simulink model "case9"  (R2024b)
settings: Solver=FixedStepAuto  StartTime=0  StopTime=1  FixedStep=1e-7  RelTol=1e-3
values from neighbouring files (symbols this model uses):
  SG_D_1_D = 0.01056    [IEEE9_case_parameters.m]    (also in case1_parameters.m; case2_parameters.m; case3_parameters.m; case4_parameters.m)
  SG_D_1_EnableSaturation = 0    [IEEE9_case_parameters.m]    (also in case1_parameters.m; case2_parameters.m; case3_parameters.m; case4_parameters.m)
  SG_D_1_f0 = 60    [IEEE9_case_parameters.m]    (also in case1_parameters.m; case2_parameters.m; case3_parameters.m; case4_parameters.m)
  SG_D_1_H = 7.5    [IEEE9_case_parameters.m]    (also in case1_parameters.m; case2_parameters.m; case3_parameters.m; case4_parameters.m)
  SG_D_1_K_A = 20    [IEEE9_case_parameters.m]    (also in case1_parameters.m; case2_parameters.m; case3_parameters.m; case4_parameters.m)
  SG_D_1_K_E = 1.000000e+1    (= 10)    [IEEE9_case_parameters.m]    (also in case1_parameters.m; case2_parameters.m; case3_parameters.m; case4_parameters.m)
  SG_D_1_K_F = 2.363    [IEEE9_case_parameters.m]    (also in case1_parameters.m; case2_parameters.m; case3_parameters.m; case4_parameters.m)
  SG_D_1_K_s = 0.5    [IEEE9_case_parameters.m]    (also in case1_parameters.m = 5; case2_parameters.m = 5; case3_parameters.m = 5; case4_parameters.m = 5)
  SG_D_1_R_a = 0.001088    [IEEE9_case_parameters.m]    (also in case1_parameters.m; case2_parameters.m; case3_parameters.m; case4_parameters.m)
  SG_D_1_S_A = 1    [IEEE9_case_parameters.m]    (also in case1_parameters.m; case2_parameters.m; case3_parameters.m; case4_parameters.m)
  SG_D_1_S_B = 0.103    [IEEE9_case_parameters.m]    (also in case1_parameters.m; case2_parameters.m; case3_parameters.m; case4_parameters.m)
  SG_D_1_S_N = 10.659857    [IEEE9_case_parameters.m]    (also in case1_parameters.m; case2_parameters.m; case3_parameters.m; case4_parameters.m)
  SG_D_1_SpeedPara = 200    [IEEE9_case_parameters.m]    (also in case1_parameters.m; case2_parameters.m; case3_parameters.m; case4_parameters.m)
  SG_D_1_T_0 = 0.720173    [IEEE9_case_parameters.m]    (also in case1_parameters.m = 0.755522; case2_parameters.m = 0.808931; case3_parameters.m = 0.869402; case4_parameters.m = 0.729316)
  SG_D_1_T_1 = 0.3    [IEEE9_case_parameters.m]    (also in case1_parameters.m; case2_parameters.m; case3_parameters.m; case4_parameters.m)
  SG_D_1_T_2 = 0.05    [IEEE9_case_parameters.m]    (also in case1_parameters.m; case2_parameters.m; case3_parameters.m; case4_parameters.m)
  SG_D_1_T_3 = 0.02    [IEEE9_case_parameters.m]    (also in case1_parameters.m; case2_parameters.m; case3_parameters.m; case4_parameters.m)
  SG_D_1_T_4 = 0.005    [IEEE9_case_parameters.m]    (also in case1_parameters.m; case2_parameters.m; case3_parameters.m; case4_parameters.m)
  SG_D_1_T_A = 0.02    [IEEE9_case_parameters.m]    (also in case1_parameters.m; case2_parameters.m; case3_parameters.m; case4_parameters.m)
  SG_D_1_T_dd = 8.000000e+0    (= 8)    [IEEE9_case_parameters.m]    (also in case1_parameters.m; case2_parameters.m; case3_parameters.m; case4_parameters.m)
  SG_D_1_T_ddd = 0.04    [IEEE9_case_parameters.m]    (also in case1_parameters.m; case2_parameters.m; case3_parameters.m; case4_parameters.m)
  SG_D_1_T_E = 0.314    [IEEE9_case_parameters.m]    (also in case1_parameters.m; case2_parameters.m; case3_parameters.m; case4_parameters.m)
  SG_D_1_T_F = 0.35    [IEEE9_case_parameters.m]    (also in case1_parameters.m; case2_parameters.m; case3_parameters.m; case4_parameters.m)
  SG_D_1_T_qd = 0.8    [IEEE9_case_parameters.m]    (also in case1_parameters.m; case2_parameters.m; case3_parameters.m; case4_parameters.m)
  SG_D_1_T_qdd = 0.02    [IEEE9_case_parameters.m]    (also in case1_parameters.m; case2_parameters.m; case3_parameters.m; case4_parameters.m)
  SG_D_1_T_speed = 0.1    [IEEE9_case_parameters.m]    (also in case1_parameters.m = 200; case2_parameters.m = 200; case3_parameters.m = 200; case4_parameters.m = 200)
  SG_D_1_T_w = 0.5    [IEEE9_case_parameters.m]    (also in case1_parameters.m; case2_parameters.m; case3_parameters.m; case4_parameters.m)
  SG_D_1_V_ref = 1.990276    [IEEE9_case_parameters.m]    (also in case1_parameters.m = 2.042296; case2_parameters.m = 2.051388; case3_parameters.m = 2.089584; case4_parameters.m = 2.01845)
  SG_D_1_w_ref = 376.991118    [IEEE9_case_parameters.m]    (also in case1_parameters.m; case2_parameters.m; case3_parameters.m; case4_parameters.m)
  SG_D_1_wb = 6.000000e+1    (= 60)    [IEEE9_case_parameters.m]    (also in case1_parameters.m; case2_parameters.m; case3_parameters.m; case4_parameters.m)
  SG_D_1_x_d = 1.9    [IEEE9_case_parameters.m]    (also in case1_parameters.m; case2_parameters.m; case3_parameters.m; case4_parameters.m)
  SG_D_1_x_dd = 0.302    [IEEE9_case_parameters.m]    (also in case1_parameters.m; case2_parameters.m; case3_parameters.m; case4_parameters.m)
  SG_D_1_x_ddd = 0.204    [IEEE9_case_parameters.m]    (also in case1_parameters.m; case2_parameters.m; case3_parameters.m; case4_parameters.m)
  SG_D_1_x_l = 0.05    [IEEE9_case_parameters.m]    (also in case1_parameters.m; case2_parameters.m; case3_parameters.m; case4_parameters.m)
  SG_D_1_x_q = 1.3    [IEEE9_case_parameters.m]    (also in case1_parameters.m; case2_parameters.m; case3_parameters.m; case4_parameters.m)
  SG_D_1_x_qd = 0.5    [IEEE9_case_parameters.m]    (also in case1_parameters.m; case2_parameters.m; case3_parameters.m; case4_parameters.m)
  SG_D_1_x_qdd = 0.3    [IEEE9_case_parameters.m]    (also in case1_parameters.m; case2_parameters.m; case3_parameters.m; case4_parameters.m)
  SG_D_2_D = 0.02    [IEEE9_case_parameters.m]    (also in case1_parameters.m; case2_parameters.m; case3_parameters.m; case4_parameters.m)
  SG_D_2_EnableSaturation = 0    [IEEE9_case_parameters.m]    (also in case1_parameters.m; case2_parameters.m; case3_parameters.m; case4_parameters.m)
  SG_D_2_f0 = 60    [IEEE9_case_parameters.m]    (also in case1_parameters.m; case2_parameters.m; case3_parameters.m; case4_parameters.m)
  SG_D_2_H = 8.000000e+0    (= 8)    [IEEE9_case_parameters.m]    (also in case1_parameters.m; case2_parameters.m; case3_parameters.m; case4_parameters.m)
  SG_D_2_K_A = 20    [IEEE9_case_parameters.m]    (also in case1_parameters.m; case2_parameters.m; case3_parameters.m; case4_parameters.m)
  SG_D_2_K_E = 1.000000e+1    (= 10)    [IEEE9_case_parameters.m]    (also in case1_parameters.m; case2_parameters.m; case3_parameters.m; case4_parameters.m)
  SG_D_2_K_F = 2.363    [IEEE9_case_parameters.m]    (also in case1_parameters.m; case2_parameters.m; case3_parameters.m; case4_parameters.m)
  SG_D_2_K_s = 0.5    [IEEE9_case_parameters.m]    (also in case1_parameters.m = 4; case2_parameters.m = 4; case3_parameters.m = 4; case4_parameters.m = 4)
  SG_D_2_R_a = 0.001088    [IEEE9_case_parameters.m]    (also in case1_parameters.m; case2_parameters.m; case3_parameters.m; case4_parameters.m)
  SG_D_2_S_A = 1    [IEEE9_case_parameters.m]    (also in case1_parameters.m; case2_parameters.m; case3_parameters.m; case4_parameters.m)
  SG_D_2_S_B = 0.103    [IEEE9_case_parameters.m]    (also in case1_parameters.m; case2_parameters.m; case3_parameters.m; case4_parameters.m)
  SG_D_2_S_N = 10.659857    [IEEE9_case_parameters.m]    (also in case1_parameters.m; case2_parameters.m; case3_parameters.m; case4_parameters.m)
  SG_D_2_SpeedPara = 200    [IEEE9_case_parameters.m]    (also in case1_parameters.m; case2_parameters.m; case3_parameters.m; case4_parameters.m)
  SG_D_2_T_0 = 1.632913    [IEEE9_case_parameters.m]    (also in case1_parameters.m = 1.632925; case2_parameters.m = 1.632915; case3_parameters.m = 1.632914; case4_parameters.m = 1.632927)
  SG_D_2_T_1 = 0.2    [IEEE9_case_parameters.m]    (also in case1_parameters.m; case2_parameters.m; case3_parameters.m; case4_parameters.m)
  SG_D_2_T_2 = 0.05    [IEEE9_case_parameters.m]    (also in case1_parameters.m; case2_parameters.m; case3_parameters.m; case4_parameters.m)
  SG_D_2_T_3 = 0.02    [IEEE9_case_parameters.m]    (also in case1_parameters.m; case2_parameters.m; case3_parameters.m; case4_parameters.m)
  SG_D_2_T_4 = 0.005    [IEEE9_case_parameters.m]    (also in case1_parameters.m; case2_parameters.m; case3_parameters.m; case4_parameters.m)
  SG_D_2_T_A = 0.02    [IEEE9_case_parameters.m]    (also in case1_parameters.m; case2_parameters.m; case3_parameters.m; case4_parameters.m)
  SG_D_2_T_dd = 7.9    [IEEE9_case_parameters.m]    (also in case1_parameters.m; case2_parameters.m; case3_parameters.m; case4_parameters.m)
  SG_D_2_T_ddd = 0.04    [IEEE9_case_parameters.m]    (also in case1_parameters.m; case2_parameters.m; case3_parameters.m; case4_parameters.m)
  SG_D_2_T_E = 0.314    [IEEE9_case_parameters.m]    (also in case1_parameters.m; case2_parameters.m; case3_parameters.m; case4_parameters.m)
  SG_D_2_T_F = 0.35    [IEEE9_case_parameters.m]    (also in case1_parameters.m; case2_parameters.m; case3_parameters.m; case4_parameters.m)
  SG_D_2_T_qd = 0.8    [IEEE9_case_parameters.m]    (also in case1_parameters.m; case2_parameters.m; case3_parameters.m; case4_parameters.m)
  SG_D_2_T_qdd = 0.015    [IEEE9_case_parameters.m]    (also in case1_parameters.m; case2_parameters.m; case3_parameters.m; case4_parameters.m)
  SG_D_2_T_speed = 0.1    [IEEE9_case_parameters.m]    (also in case1_parameters.m = 150; case2_parameters.m = 150; case3_parameters.m = 150; case4_parameters.m = 150)
  SG_D_2_T_w = 0.35    [IEEE9_case_parameters.m]    (also in case1_parameters.m; case2_parameters.m; case3_parameters.m; case4_parameters.m)
  SG_D_2_V_ref = 2.58547    [IEEE9_case_parameters.m]    (also in case1_parameters.m = 2.597896; case2_parameters.m = 2.587136; case3_parameters.m = 2.586042; case4_parameters.m = 2.599679)
  SG_D_2_w_ref = 376.991118    [IEEE9_case_parameters.m]    (also in case1_parameters.m; case2_parameters.m; case3_parameters.m; case4_parameters.m)
  SG_D_2_wb = 6.000000e+1    (= 60)    [IEEE9_case_parameters.m]    (also in case1_parameters.m; case2_parameters.m; case3_parameters.m; case4_parameters.m)
  SG_D_2_x_d = 1.8    [IEEE9_case_parameters.m]    (also in case1_parameters.m; case2_parameters.m; case3_parameters.m; case4_parameters.m)
  SG_D_2_x_dd = 0.302    [IEEE9_case_parameters.m]    (also in case1_parameters.m; case2_parameters.m; case3_parameters.m; case4_parameters.m)
  SG_D_2_x_ddd = 0.204    [IEEE9_case_parameters.m]    (also in case1_parameters.m; case2_parameters.m; case3_parameters.m; case4_parameters.m)
  SG_D_2_x_l = 0.05    [IEEE9_case_parameters.m]    (also in case1_parameters.m; case2_parameters.m; case3_parameters.m; case4_parameters.m)
  SG_D_2_x_q = 1.25    [IEEE9_case_parameters.m]    (also in case1_parameters.m; case2_parameters.m; case3_parameters.m; case4_parameters.m)
  SG_D_2_x_qd = 0.5    [IEEE9_case_parameters.m]    (also in case1_parameters.m; case2_parameters.m; case3_parameters.m; case4_parameters.m)
  SG_D_2_x_qdd = 0.3    [IEEE9_case_parameters.m]    (also in case1_parameters.m; case2_parameters.m; case3_parameters.m; case4_parameters.m)
  SG_D_3_D = 0.02    [IEEE9_case_parameters.m]    (also in case1_parameters.m; case2_parameters.m; case3_parameters.m; case4_parameters.m)
  SG_D_3_EnableSaturation = 0    [IEEE9_case_parameters.m]    (also in case1_parameters.m; case2_parameters.m; case3_parameters.m; case4_parameters.m)
  SG_D_3_f0 = 60    [IEEE9_case_parameters.m]    (also in case1_parameters.m; case2_parameters.m; case3_parameters.m; case4_parameters.m)
  SG_D_3_H = 7.7    [IEEE9_case_parameters.m]    (also in case1_parameters.m; case2_parameters.m; case3_parameters.m; case4_parameters.m)
  SG_D_3_K_A = 20    [IEEE9_case_parameters.m]    (also in case1_parameters.m; case2_parameters.m; case3_parameters.m; case4_parameters.m)
  SG_D_3_K_E = 1.000000e+1    (= 10)    [IEEE9_case_parameters.m]    (also in case1_parameters.m; case2_parameters.m; case3_parameters.m; case4_parameters.m)
  SG_D_3_K_F = 2.363    [IEEE9_case_parameters.m]    (also in case1_parameters.m; case2_parameters.m; case3_parameters.m; case4_parameters.m)
  SG_D_3_K_s = 0.2    [IEEE9_case_parameters.m]    (also in case1_parameters.m = 2; case2_parameters.m = 2; case3_parameters.m = 2; case4_parameters.m = 2)
  SG_D_3_R_a = 0.001088    [IEEE9_case_parameters.m]    (also in case1_parameters.m; case2_parameters.m; case3_parameters.m; case4_parameters.m)
  SG_D_3_S_A = 1    [IEEE9_case_parameters.m]    (also in case1_parameters.m; case2_parameters.m; case3_parameters.m; case4_parameters.m)
  SG_D_3_S_B = 0.103    [IEEE9_case_parameters.m]    (also in case1_parameters.m; case2_parameters.m; case3_parameters.m; case4_parameters.m)
  SG_D_3_S_N = 10.659857    [IEEE9_case_parameters.m]    (also in case1_parameters.m; case2_parameters.m; case3_parameters.m; case4_parameters.m)
  SG_D_3_SpeedPara = 200    [IEEE9_case_parameters.m]    (also in case1_parameters.m; case2_parameters.m; case3_parameters.m; case4_parameters.m)
  SG_D_3_T_0 = 0.850788    [IEEE9_case_parameters.m]    (also in case1_parameters.m = 0.850786; case2_parameters.m = 0.850787; case3_parameters.m; case4_parameters.m = 0.850786)
  SG_D_3_T_1 = 0.2    [IEEE9_case_parameters.m]    (also in case1_parameters.m; case2_parameters.m; case3_parameters.m; case4_parameters.m)
  SG_D_3_T_2 = 0.05    [IEEE9_case_parameters.m]    (also in case1_parameters.m; case2_parameters.m; case3_parameters.m; case4_parameters.m)
  SG_D_3_T_3 = 0.02    [IEEE9_case_parameters.m]    (also in case1_parameters.m; case2_parameters.m; case3_parameters.m; case4_parameters.m)
  SG_D_3_T_4 = 0.005    [IEEE9_case_parameters.m]    (also in case1_parameters.m; case2_parameters.m; case3_parameters.m; case4_parameters.m)
  SG_D_3_T_A = 0.02    [IEEE9_case_parameters.m]    (also in case1_parameters.m; case2_parameters.m; case3_parameters.m; case4_parameters.m)
  SG_D_3_T_dd = 8.1    [IEEE9_case_parameters.m]    (also in case1_parameters.m; case2_parameters.m; case3_parameters.m; case4_parameters.m)
  SG_D_3_T_ddd = 0.04    [IEEE9_case_parameters.m]    (also in case1_parameters.m; case2_parameters.m; case3_parameters.m; case4_parameters.m)
  SG_D_3_T_E = 0.314    [IEEE9_case_parameters.m]    (also in case1_parameters.m; case2_parameters.m; case3_parameters.m; case4_parameters.m)
  SG_D_3_T_F = 0.35    [IEEE9_case_parameters.m]    (also in case1_parameters.m; case2_parameters.m; case3_parameters.m; case4_parameters.m)
  SG_D_3_T_qd = 0.8    [IEEE9_case_parameters.m]    (also in case1_parameters.m; case2_parameters.m; case3_parameters.m; case4_parameters.m)
  SG_D_3_T_qdd = 0.015    [IEEE9_case_parameters.m]    (also in case1_parameters.m; case2_parameters.m; case3_parameters.m; case4_parameters.m)
  SG_D_3_T_speed = 0.1    [IEEE9_case_parameters.m]    (also in case1_parameters.m = 180; case2_parameters.m = 180; case3_parameters.m = 180; case4_parameters.m = 180)
  SG_D_3_T_w = 0.4    [IEEE9_case_parameters.m]    (also in case1_parameters.m; case2_parameters.m; case3_parameters.m; case4_parameters.m)
  SG_D_3_V_ref = 1.892727    [IEEE9_case_parameters.m]    (also in case1_parameters.m = 1.906439; case2_parameters.m = 1.895535; case3_parameters.m = 1.892105; case4_parameters.m = 1.906598)
  SG_D_3_w_ref = 376.991118    [IEEE9_case_parameters.m]    (also in case1_parameters.m; case2_parameters.m; case3_parameters.m; case4_parameters.m)
  SG_D_3_wb = 6.000000e+1    (= 60)    [IEEE9_case_parameters.m]    (also in case1_parameters.m; case2_parameters.m; case3_parameters.m; case4_parameters.m)
  SG_D_3_x_d = 1.85    [IEEE9_case_parameters.m]    (also in case1_parameters.m; case2_parameters.m; case3_parameters.m; case4_parameters.m)
  SG_D_3_x_dd = 0.302    [IEEE9_case_parameters.m]    (also in case1_parameters.m; case2_parameters.m; case3_parameters.m; case4_parameters.m)
  SG_D_3_x_ddd = 0.204    [IEEE9_case_parameters.m]    (also in case1_parameters.m; case2_parameters.m; case3_parameters.m; case4_parameters.m)
  SG_D_3_x_l = 0.05    [IEEE9_case_parameters.m]    (also in case1_parameters.m; case2_parameters.m; case3_parameters.m; case4_parameters.m)
  SG_D_3_x_q = 1.2    [IEEE9_case_parameters.m]    (also in case1_parameters.m; case2_parameters.m; case3_parameters.m; case4_parameters.m)
  SG_D_3_x_qd = 0.5    [IEEE9_case_parameters.m]    (also in case1_parameters.m; case2_parameters.m; case3_parameters.m; case4_parameters.m)
  SG_D_3_x_qdd = 0.3    [IEEE9_case_parameters.m]    (also in case1_parameters.m; case2_parameters.m; case3_parameters.m; case4_parameters.m)
(part 7 of 12)

== system case9/Apparatus/SG_D_1/i_q_SG_D_1_block ==
  note: i_q_SG_D_1 in case9
      | $-\frac{\sin\left(\theta _{\mathrm{SG},D,1}\right)\,\left(\psi _{q,\mathrm{SG},D,1}+\frac{\psi _{\mathrm{gq},\mathrm{SG},D,1}\,\left(x_{l}-x_{\mathrm{qdd}}\right)}{x_{l}-x_{\mathrm{qd}}}+\frac{\psi _{\mathrm{kq},\mathrm{SG},D,1}\,\left(x_{\mathrm{qd}}-x_{\mathrm{qdd}}\right)}{x_{l}-x_{\mathrm{qd}}}\right)}{x_{\mathrm{qdd}}}-\frac{\cos\left(\theta _{\mathrm{SG},D,1}\right)\,\left(\frac{\psi _{\mathrm{1d},\mathrm{SG},D,1}\,\left(x_{\mathrm{dd}}-x_{\mathrm{ddd}}\right)}{x_{\mathrm{dd}}-x_{l}}-\psi _{d,\mathrm{SG},D,1}+\frac{\psi _{\mathrm{fd},\mathrm{SG},D,1}\,\left(x_{\mathrm{ddd}}-x_{l}\right)}{x_{\mathrm{dd}}-x_{l}}\right)}{x_{\mathrm{ddd}}}$
      | Automatically generated on 2025-10-31 19:34:49 .
  State_psi_gq_SG_D_1_092c5 : Inport
  State_psi_kq_SG_D_1_97f5f : Inport  Port=2
  State_psi_q_SG_D_1_fdadd : Inport  Port=3
  State_theta_SG_D_1_3c1fa : Inport  Port=4
  State_psi_1d_SG_D_1_7b40d : Inport  Port=5
  State_psi_d_SG_D_1_0e386 : Inport  Port=6
  State_psi_fd_SG_D_1_9fe64 : Inport  Port=7
  State_theta_SG_D_1_71fb6 : Inport  Port=8
  Add_0017d : Sum
  Add_35a64 : Sum
  Add_56630 : Sum
  Add_62db7 : Sum
  Add_95d78 : Sum
  Add_e1f2e : Sum
  Constant_-1_14a26 : Constant  Value=-1
  Constant_-1_1cd36 : Constant  Value=-1
  Constant_-1_24052 : Constant  Value=-1
  Constant_-1_72e90 : Constant  Value=-1
  Constant_-1_8fd2e : Constant  Value=-1
  Constant_x_dd_843a6 : Constant  Value=x_dd
  Constant_x_dd_8e74f : Constant  Value=x_dd
  Constant_x_dd_e3151 : Constant  Value=x_dd
  Constant_x_ddd_51e8b : Constant  Value=x_ddd
  Constant_x_ddd_cca8e : Constant  Value=x_ddd
  Constant_x_ddd_d6eda : Constant  Value=x_ddd
  Constant_x_l_3e9e8 : Constant  Value=x_l
  Constant_x_l_9dea0 : Constant  Value=x_l
  Constant_x_l_a6233 : Constant  Value=x_l
  Constant_x_l_c84a1 : Constant  Value=x_l
  Constant_x_l_c867c : Constant  Value=x_l
  Constant_x_l_f552f : Constant  Value=x_l
  Constant_x_qd_56b92 : Constant  Value=x_qd
  Constant_x_qd_58631 : Constant  Value=x_qd
  Constant_x_qd_adad9 : Constant  Value=x_qd
  Constant_x_qdd_01789 : Constant  Value=x_qdd
  Constant_x_qdd_72f85 : Constant  Value=x_qdd
  Constant_x_qdd_ff6ca : Constant  Value=x_qdd
  Divide_65d14 : Product  Inputs=*/
  Divide_84916 : Product  Inputs=*/
  Divide_a2796 : Product  Inputs=*/
  Divide_a496a : Product  Inputs=*/
  Divide_bf3d1 : Product  Inputs=*/
  Divide_d6104 : Product  Inputs=*/
  MathFunc_cos_5e1d4 : Trigonometry  Operator=cos
  MathFunc_sin_468db : Trigonometry
  Product_13cd1 : Product
  Product_232ad : Product
  Product_41f3d : Product
  Product_456f6 : Product
  Product_4694f : Product
  Product_4cb2c : Product
  Product_83cb5 : Product
  Product_a6406 : Product
  Product_a9c33 : Product
  Product_d6079 : Product
  Product_f9405 : Product
  Subtract_3022c : Sum  Inputs=+-
  Subtract_3886e : Sum  Inputs=+-
  Subtract_5dabf : Sum  Inputs=+-
  Subtract_96f7c : Sum  Inputs=+-
  Subtract_9b1aa : Sum  Inputs=+-
  Subtract_e0046 : Sum  Inputs=+-
  Subtract_ea4b7 : Sum  Inputs=+-
  Blockout_i_q_SG_D_1_cd846 : Outport
  wires:
  State_theta_SG_D_1_71fb6/1 -> MathFunc_cos_5e1d4/1
  State_psi_fd_SG_D_1_9fe64/1 -> Product_f9405/1
  Constant_-1_72e90/1 -> Product_a6406/1
  Constant_x_l_c867c/1 -> Product_a6406/2
  Subtract_5dabf/1 -> Product_f9405/2
  Constant_x_l_9dea0/1 -> Subtract_9b1aa/2
  Product_a6406/1 -> Add_0017d/1
  Constant_x_qdd_ff6ca/1 -> Add_0017d/2
  Constant_x_qd_adad9/1 -> Subtract_e0046/1
  Constant_x_qdd_72f85/1 -> Divide_65d14/2
  MathFunc_sin_468db/1 -> Product_13cd1/2
  Constant_-1_8fd2e/1 -> Product_83cb5/1
  Constant_x_qdd_01789/1 -> Subtract_e0046/2
  Add_56630/1 -> Product_4694f/2
  Product_456f6/1 -> Divide_84916/1
  Constant_x_l_f552f/1 -> Product_83cb5/2
  Constant_-1_14a26/1 -> Product_232ad/1
  Constant_x_l_3e9e8/1 -> Product_232ad/2
  State_psi_gq_SG_D_1_092c5/1 -> Product_456f6/1
  Add_0017d/1 -> Product_456f6/2
  Divide_a496a/1 -> Add_e1f2e/1
  Product_83cb5/1 -> Add_35a64/1
  Divide_65d14/1 -> Add_95d78/1
  Constant_x_qd_56b92/1 -> Add_35a64/2
  State_psi_kq_SG_D_1_97f5f/1 -> Product_4cb2c/1
  Add_e1f2e/1 -> Subtract_96f7c/1
  Subtract_e0046/1 -> Product_4cb2c/2
  Divide_84916/1 -> Subtract_3022c/1
  Add_35a64/1 -> Divide_84916/2
  Product_232ad/1 -> Add_62db7/1
  Constant_x_qd_58631/1 -> Add_62db7/2
  Constant_-1_1cd36/1 -> Product_a9c33/1
  MathFunc_cos_5e1d4/1 -> Product_d6079/2
  Product_f9405/1 -> Divide_d6104/1
  State_psi_1d_SG_D_1_7b40d/1 -> Product_a9c33/2
  Constant_x_l_c84a1/1 -> Subtract_3886e/2
  Constant_x_dd_e3151/1 -> Subtract_ea4b7/1
  Divide_d6104/1 -> Subtract_96f7c/2
  Constant_x_ddd_d6eda/1 -> Subtract_ea4b7/2
  Product_d6079/1 -> Divide_bf3d1/1
  Product_4cb2c/1 -> Divide_a2796/1
  Product_a9c33/1 -> Product_41f3d/1
  Add_62db7/1 -> Divide_a2796/2
  Subtract_ea4b7/1 -> Product_41f3d/2
  State_psi_d_SG_D_1_0e386/1 -> Add_e1f2e/2
  Constant_x_dd_8e74f/1 -> Subtract_9b1aa/1
  Constant_x_ddd_cca8e/1 -> Subtract_5dabf/1
  Constant_x_l_a6233/1 -> Subtract_5dabf/2
  Divide_bf3d1/1 -> Add_95d78/2
  Divide_a2796/1 -> Subtract_3022c/2
  State_theta_SG_D_1_3c1fa/1 -> MathFunc_sin_468db/1
  Product_41f3d/1 -> Divide_a496a/1
  Subtract_9b1aa/1 -> Divide_a496a/2
  Constant_x_dd_843a6/1 -> Subtract_3886e/1
  Subtract_3022c/1 -> Add_56630/1
  State_psi_q_SG_D_1_fdadd/1 -> Add_56630/2
  Subtract_3886e/1 -> Divide_d6104/2
  Subtract_96f7c/1 -> Product_d6079/1
  Constant_-1_24052/1 -> Product_4694f/1
  Product_4694f/1 -> Product_13cd1/1
  Product_13cd1/1 -> Divide_65d14/1
  Constant_x_ddd_51e8b/1 -> Divide_bf3d1/2
  Add_95d78/1 -> Blockout_i_q_SG_D_1_cd846/1

== system case9/Apparatus/SG_D_1/theta_SG_D_1_out_block ==
  note: theta_SG_D_1_out in case9
      | $\theta _{\mathrm{SG},D,1}$
      | Automatically generated on 2025-10-31 19:34:50 .
  State_theta_SG_D_1_b223f : Inport
  Blockout_theta_SG_D_1_out_ac5bf : Outport
  wires:
  State_theta_SG_D_1_b223f/1 -> Blockout_theta_SG_D_1_out_ac5bf/1

== system case9/Apparatus/SG_D_1/w_SG_D_1_out_block ==
  note: w_SG_D_1_out in case9
      | $w_{\mathrm{SG},D,1}$
      | Automatically generated on 2025-10-31 19:34:50 .
  State_w_SG_D_1_3e49a : Inport
  Blockout_w_SG_D_1_out_45494 : Outport
  wires:
  State_w_SG_D_1_3e49a/1 -> Blockout_w_SG_D_1_out_45494/1

== system case9/Apparatus/SG_D_2/T_e_SG_D_2_block ==
  note: T_e_SG_D_2 in case9
      | $-\frac{\psi _{d,\mathrm{SG},D,2}\,\left(\psi _{q,\mathrm{SG},D,2}+\frac{\psi _{\mathrm{gq},\mathrm{SG},D,2}\,\left(x_{l}-x_{\mathrm{qdd}}\right)}{x_{l}-x_{\mathrm{qd}}}+\frac{\psi _{\mathrm{kq},\mathrm{SG},D,2}\,\left(x_{\mathrm{qd}}-x_{\mathrm{qdd}}\right)}{x_{l}-x_{\mathrm{qd}}}\right)}{x_{\mathrm{qdd}}}-\frac{\psi _{q,\mathrm{SG},D,2}\,\left(\frac{\psi _{\mathrm{1d},\mathrm{SG},D,2}\,\left(x_{\mathrm{dd}}-x_{\mathrm{ddd}}\right)}{x_{\mathrm{dd}}-x_{l}}-\psi _{d,\mathrm{SG},D,2}+\frac{\psi _{\mathrm{fd},\mathrm{SG},D,2}\,\left(x_{\mathrm{ddd}}-x_{l}\right)}{x_{\mathrm{dd}}-x_{l}}\right)}{x_{\mathrm{ddd}}}$
      | Automatically generated on 2025-10-31 19:35:08 .
  State_psi_d_SG_D_2_9606a : Inport
  State_psi_gq_SG_D_2_f0a68 : Inport  Port=2
  State_psi_kq_SG_D_2_17e3d : Inport  Port=3
  State_psi_q_SG_D_2_a73d1 : Inport  Port=4
  State_psi_q_SG_D_2_2dc20 : Inport  Port=5
  State_psi_1d_SG_D_2_dfc50 : Inport  Port=6
  State_psi_d_SG_D_2_7cb77 : Inport  Port=7
  State_psi_fd_SG_D_2_946fe : Inport  Port=8
  Add_0b222 : Sum
  Add_30e81 : Sum
  Add_8b206 : Sum
  Add_d85b4 : Sum
  Add_e0a82 : Sum
  Add_ed19d : Sum
  Constant_-1_3a2ab : Constant  Value=-1
  Constant_-1_81492 : Constant  Value=-1
  Constant_-1_89beb : Constant  Value=-1
  Constant_-1_b1e92 : Constant  Value=-1
  Constant_-1_c9ed8 : Constant  Value=-1
  Constant_x_dd_50243 : Constant  Value=x_dd
  Constant_x_dd_be71b : Constant  Value=x_dd
  Constant_x_dd_dd49a : Constant  Value=x_dd
  Constant_x_ddd_2d22c : Constant  Value=x_ddd
  Constant_x_ddd_b2247 : Constant  Value=x_ddd
  Constant_x_ddd_d3b5a : Constant  Value=x_ddd
  Constant_x_l_1576d : Constant  Value=x_l
  Constant_x_l_72a63 : Constant  Value=x_l
  Constant_x_l_91dea : Constant  Value=x_l
  Constant_x_l_b4de2 : Constant  Value=x_l
  Constant_x_l_bb09d : Constant  Value=x_l
  Constant_x_l_e80c1 : Constant  Value=x_l
  Constant_x_qd_20bdd : Constant  Value=x_qd
  Constant_x_qd_9a586 : Constant  Value=x_qd
  Constant_x_qd_bcee2 : Constant  Value=x_qd
  Constant_x_qdd_146fc : Constant  Value=x_qdd
  Constant_x_qdd_28a0e : Constant  Value=x_qdd
  Constant_x_qdd_c7836 : Constant  Value=x_qdd
  Divide_1415d : Product  Inputs=*/
  Divide_24622 : Product  Inputs=*/
  Divide_4fb71 : Product  Inputs=*/
  Divide_6dd3b : Product  Inputs=*/
  Divide_801a8 : Product  Inputs=*/
  Divide_a4770 : Product  Inputs=*/
  Product_10174 : Product
  Product_280fc : Product
  Product_3044b : Product
  Product_3eab5 : Product
  Product_600d6 : Product
  Product_6735f : Product
  Product_77108 : Product
  Product_78fb9 : Product
  Product_8289b : Product
  Product_dbfcd : Product
  Product_e661d : Product
  Subtract_1d9de : Sum  Inputs=+-
  Subtract_55562 : Sum  Inputs=+-
  Subtract_635aa : Sum  Inputs=+-
  Subtract_661d1 : Sum  Inputs=+-
  Subtract_7ba2e : Sum  Inputs=+-
  Subtract_cacd5 : Sum  Inputs=+-
  Subtract_d9381 : Sum  Inputs=+-
  Blockout_T_e_SG_D_2_742ed : Outport
  wires:
  Constant_-1_3a2ab/1 -> Product_10174/1
  Divide_801a8/1 -> Subtract_1d9de/1
  Constant_-1_c9ed8/1 -> Product_8289b/1
  Constant_x_l_91dea/1 -> Product_8289b/2
  Constant_x_qd_20bdd/1 -> Subtract_661d1/1
  Product_600d6/1 -> Divide_801a8/1
  Product_8289b/1 -> Add_ed19d/1
  Divide_24622/1 -> Subtract_55562/2
  Constant_x_qdd_28a0e/1 -> Subtract_661d1/2
  Constant_x_qdd_146fc/1 -> Divide_6dd3b/2
  Constant_x_ddd_b2247/1 -> Subtract_7ba2e/2
  Constant_x_qdd_c7836/1 -> Add_ed19d/2
  Constant_x_l_b4de2/1 -> Product_10174/2
  Constant_-1_b1e92/1 -> Product_e661d/1
  Constant_x_l_bb09d/1 -> Product_e661d/2
  Constant_-1_89beb/1 -> Product_dbfcd/1
  State_psi_1d_SG_D_2_dfc50/1 -> Product_dbfcd/2
  Constant_x_dd_50243/1 -> Subtract_7ba2e/1
  Divide_4fb71/1 -> Subtract_1d9de/2
  State_psi_gq_SG_D_2_f0a68/1 -> Product_600d6/1
  Add_ed19d/1 -> Product_600d6/2
  Subtract_1d9de/1 -> Add_e0a82/1
  Constant_x_dd_dd49a/1 -> Subtract_d9381/1
  Product_10174/1 -> Add_d85b4/1
  Product_3eab5/1 -> Product_78fb9/1
  Constant_x_qd_9a586/1 -> Add_d85b4/2
  State_psi_kq_SG_D_2_17e3d/1 -> Product_280fc/1
  Subtract_661d1/1 -> Product_280fc/2
  Product_e661d/1 -> Add_8b206/1
  State_psi_q_SG_D_2_2dc20/1 -> Product_6735f/1
  Constant_x_qd_bcee2/1 -> Add_8b206/2
  Product_dbfcd/1 -> Product_77108/1
  Divide_1415d/1 -> Add_30e81/2
  Subtract_7ba2e/1 -> Product_77108/2
  Constant_x_l_1576d/1 -> Subtract_d9381/2
  Constant_x_ddd_d3b5a/1 -> Subtract_635aa/1
  Constant_x_dd_be71b/1 -> Subtract_cacd5/1
  Constant_x_l_e80c1/1 -> Subtract_635aa/2
  Add_30e81/1 -> Blockout_T_e_SG_D_2_742ed/1
  Add_d85b4/1 -> Divide_801a8/2
  Product_280fc/1 -> Divide_4fb71/1
  Product_78fb9/1 -> Divide_6dd3b/1
  State_psi_d_SG_D_2_9606a/1 -> Product_3eab5/2
  Add_8b206/1 -> Divide_4fb71/2
  Product_77108/1 -> Divide_a4770/1
  Subtract_d9381/1 -> Divide_a4770/2
  Constant_x_l_72a63/1 -> Subtract_cacd5/2
  State_psi_fd_SG_D_2_946fe/1 -> Product_3044b/1
  Constant_x_ddd_2d22c/1 -> Divide_1415d/2
  Product_6735f/1 -> Divide_1415d/1
  Subtract_635aa/1 -> Product_3044b/2
  Divide_a4770/1 -> Add_0b222/1
  State_psi_d_SG_D_2_7cb77/1 -> Add_0b222/2
  Add_0b222/1 -> Subtract_55562/1
  Product_3044b/1 -> Divide_24622/1
  Subtract_cacd5/1 -> Divide_24622/2
  Constant_-1_81492/1 -> Product_3eab5/1
  State_psi_q_SG_D_2_a73d1/1 -> Add_e0a82/2
  Add_e0a82/1 -> Product_78fb9/2
  Subtract_55562/1 -> Product_6735f/2
  Divide_6dd3b/1 -> Add_30e81/1

== system case9/Apparatus/SG_D_2/d_E_fd_SG_D_2_block ==
  note: d_E_fd_SG_D_2 in case9
      | $\frac{V_{f,\mathrm{SG},D,2}-E_{\mathrm{fd},\mathrm{SG},D,2}\,K_{E}}{T_{E}}$
      | Automatically generated on 2025-10-31 19:35:03 .
  State_E_fd_SG_D_2_07948 : Inport
  State_V_f_SG_D_2_669e7 : Inport  Port=2
  Add_f4ac7 : Sum
  Constant_-1_f9b1f : Constant  Value=-1
  Constant_K_E_6fab2 : Constant  Value=K_E
  Constant_T_E_88b54 : Constant  Value=T_E
  Divide_66be5 : Product  Inputs=*/
  Product_e9996 : Product
  Product_f9514 : Product
  Blockout_d_E_fd_SG_D_2_d61cc : Outport
  wires:
  Constant_-1_f9b1f/1 -> Product_f9514/1
  State_E_fd_SG_D_2_07948/1 -> Product_f9514/2
  Product_f9514/1 -> Product_e9996/1
  Constant_K_E_6fab2/1 -> Product_e9996/2
  Product_e9996/1 -> Add_f4ac7/1
  Constant_T_E_88b54/1 -> Divide_66be5/2
  State_V_f_SG_D_2_669e7/1 -> Add_f4ac7/2
  Add_f4ac7/1 -> Divide_66be5/1
  Divide_66be5/1 -> Blockout_d_E_fd_SG_D_2_d61cc/1

== system case9/Apparatus/SG_D_2/d_Px_1_SG_D_2_block ==
  note: d_Px_1_SG_D_2 in case9
      | $\frac{w_{\mathrm{SG},D,2}-2\,\pi \,f_{0}}{T_{w}}-\frac{\mathrm{Px}_{1,\mathrm{SG},D,2}}{T_{w}}$
      | Automatically generated on 2025-10-31 19:35:04 .
  State_Px_1_SG_D_2_2a6d5 : Inport
  State_w_SG_D_2_4e30f : Inport  Port=2
  Add_16545 : Sum
  Add_60d76 : Sum
  Constant_-1_4fc01 : Constant  Value=-1
  Constant_-2.0_1ffa0 : Constant  Value=-2.0
  Constant_T_w_65d02 : Constant  Value=T_w
  Constant_T_w_88523 : Constant  Value=T_w
  Constant_f0_994d3 : Constant  Value=f0
  Constant_pi_80fb2 : Constant  Value=pi
  Divide_46284 : Product  Inputs=*/
  Divide_59f41 : Product  Inputs=*/
  Product_88dc0 : Product
  Product_93f5d : Product
  Product_ff1bb : Product
  Blockout_d_Px_1_SG_D_2_3bd8b : Outport
  wires:
  Constant_-2.0_1ffa0/1 -> Product_88dc0/1
  State_w_SG_D_2_4e30f/1 -> Add_16545/2
  Constant_pi_80fb2/1 -> Product_88dc0/2
  Product_88dc0/1 -> Product_93f5d/1
  Constant_f0_994d3/1 -> Product_93f5d/2
  Constant_-1_4fc01/1 -> Product_ff1bb/1
  State_Px_1_SG_D_2_2a6d5/1 -> Product_ff1bb/2
  Product_93f5d/1 -> Add_16545/1
  Product_ff1bb/1 -> Divide_59f41/1
  Constant_T_w_88523/1 -> Divide_59f41/2
  Add_16545/1 -> Divide_46284/1
  Constant_T_w_65d02/1 -> Divide_46284/2
  Divide_59f41/1 -> Add_60d76/1
  Divide_46284/1 -> Add_60d76/2
  Add_60d76/1 -> Blockout_d_Px_1_SG_D_2_3bd8b/1

== system case9/Apparatus/SG_D_2/d_Px_2_SG_D_2_block ==
  note: d_Px_2_SG_D_2 in case9
      | $\frac{\mathrm{Px}_{1,\mathrm{SG},D,2}-T_{2}\,\left(\frac{\mathrm{Px}_{1,\mathrm{SG},D,2}}{T_{w}}-\frac{w_{\mathrm{SG},D,2}-2\,\pi \,f_{0}}{T_{w}}\right)}{T_{1}}-\frac{\mathrm{Px}_{2,\mathrm{SG},D,2}}{T_{1}}$
      | Automatically generated on 2025-10-31 19:35:04 .
  State_Px_2_SG_D_2_86e60 : Inport
  State_Px_1_SG_D_2_4e267 : Inport  Port=2
  State_Px_1_SG_D_2_978be : Inport  Port=3
  State_w_SG_D_2_89dde : Inport  Port=4
  Add_48c47 : Sum
  Add_99edd : Sum
  Add_eb8be : Sum
  Add_f699f : Sum
  Constant_-1_ab6b9 : Constant  Value=-1
  Constant_-1_c94cf : Constant  Value=-1
  Constant_-2.0_40cdb : Constant  Value=-2.0
  Constant_T_1_716d8 : Constant  Value=T_1
  Constant_T_1_a99cf : Constant  Value=T_1
  Constant_T_2_16625 : Constant  Value=T_2
  Constant_T_w_ac8fd : Constant  Value=T_w
  Constant_T_w_f304a : Constant  Value=T_w
  Constant_f0_15f3b : Constant  Value=f0
  Constant_pi_b9655 : Constant  Value=pi
  Divide_105b3 : Product  Inputs=*/
  Divide_898f9 : Product  Inputs=*/
  Divide_917a9 : Product  Inputs=*/
  Divide_a144c : Product  Inputs=*/
  Product_3a2cb : Product
  Product_a1182 : Product
  Product_ba3a2 : Product
  Product_dc02d : Product
  Product_f6dda : Product
  Blockout_d_Px_2_SG_D_2_413da : Outport
  wires:
  Constant_-1_ab6b9/1 -> Product_dc02d/1
  Constant_-2.0_40cdb/1 -> Product_3a2cb/1
  Product_a1182/1 -> Add_99edd/2
  State_w_SG_D_2_89dde/1 -> Add_f699f/2
  Constant_pi_b9655/1 -> Product_3a2cb/2
  Product_3a2cb/1 -> Product_f6dda/1
  State_Px_1_SG_D_2_978be/1 -> Product_ba3a2/2
  Constant_f0_15f3b/1 -> Product_f6dda/2
  State_Px_2_SG_D_2_86e60/1 -> Product_dc02d/2
  Constant_-1_c94cf/1 -> Product_ba3a2/1
  Product_f6dda/1 -> Add_f699f/1
  Product_ba3a2/1 -> Divide_917a9/1
  Constant_T_w_ac8fd/1 -> Divide_917a9/2
  Add_f699f/1 -> Divide_a144c/1
  Constant_T_w_f304a/1 -> Divide_a144c/2
  Divide_917a9/1 -> Add_48c47/1
  Divide_a144c/1 -> Add_48c47/2
  Constant_T_2_16625/1 -> Product_a1182/1
  Add_48c47/1 -> Product_a1182/2
  State_Px_1_SG_D_2_4e267/1 -> Add_99edd/1
  Product_dc02d/1 -> Divide_898f9/1
  Constant_T_1_716d8/1 -> Divide_898f9/2
  Add_99edd/1 -> Divide_105b3/1
  Constant_T_1_a99cf/1 -> Divide_105b3/2
  Divide_898f9/1 -> Add_eb8be/1
  Divide_105b3/1 -> Add_eb8be/2
  Add_eb8be/1 -> Blockout_d_Px_2_SG_D_2_413da/1

== system case9/Apparatus/SG_D_2/d_Px_3_SG_D_2_block ==
  note: d_Px_3_SG_D_2 in case9
      | $\frac{\mathrm{Px}_{2,\mathrm{SG},D,2}+T_{4}\,\left(\frac{\mathrm{Px}_{1,\mathrm{SG},D,2}-T_{2}\,\left(\frac{\mathrm{Px}_{1,\mathrm{SG},D,2}}{T_{w}}-\frac{w_{\mathrm{SG},D,2}-2\,\pi \,f_{0}}{T_{w}}\right)}{T_{1}}-\frac{\mathrm{Px}_{2,\mathrm{SG},D,2}}{T_{1}}\right)}{T_{3}}-\frac{\mathrm{Px}_{3,\mathrm{SG},D,2}}{T_{3}}$
      | Automatically generated on 2025-10-31 19:35:05 .
  State_Px_3_SG_D_2_7c23f : Inport
  State_Px_2_SG_D_2_f11c4 : Inport  Port=2
  State_Px_2_SG_D_2_0e6bc : Inport  Port=3
  State_Px_1_SG_D_2_ff7e4 : Inport  Port=4
  State_Px_1_SG_D_2_b2a07 : Inport  Port=5
  State_w_SG_D_2_fbd3a : Inport  Port=6
  Add_1629a : Sum
  Add_41ee7 : Sum
  Add_d6f14 : Sum
  Add_dc3fb : Sum
  Add_faa06 : Sum
  Add_facde : Sum
  Constant_-1_2becf : Constant  Value=-1
  Constant_-1_4eb38 : Constant  Value=-1
  Constant_-1_71591 : Constant  Value=-1
  Constant_-2.0_141dd : Constant  Value=-2.0
  Constant_T_1_072f9 : Constant  Value=T_1
  Constant_T_1_69240 : Constant  Value=T_1
  Constant_T_2_9993e : Constant  Value=T_2
  Constant_T_3_09de0 : Constant  Value=T_3
  Constant_T_3_ac430 : Constant  Value=T_3
  Constant_T_4_abecd : Constant  Value=T_4
  Constant_T_w_13561 : Constant  Value=T_w
  Constant_T_w_8d456 : Constant  Value=T_w
  Constant_f0_dc763 : Constant  Value=f0
  Constant_pi_f2472 : Constant  Value=pi
  Divide_10a1c : Product  Inputs=*/
  Divide_4bdb1 : Product  Inputs=*/
  Divide_56502 : Product  Inputs=*/
  Divide_615c2 : Product  Inputs=*/
  Divide_8e81c : Product  Inputs=*/
  Divide_e6edd : Product  Inputs=*/
  Product_28c6e : Product
  Product_5e1a3 : Product
  Product_725a7 : Product
  Product_a6171 : Product
  Product_d0fc6 : Product
  Product_ea11b : Product
  Product_f0ef2 : Product
  Blockout_d_Px_3_SG_D_2_76e34 : Outport
  wires:
  Constant_-2.0_141dd/1 -> Product_725a7/1
  State_w_SG_D_2_fbd3a/1 -> Add_d6f14/2
  Add_1629a/1 -> Divide_4bdb1/1
  Constant_pi_f2472/1 -> Product_725a7/2
  Constant_-1_71591/1 -> Product_ea11b/1
  Product_725a7/1 -> Product_d0fc6/1
  State_Px_2_SG_D_2_0e6bc/1 -> Product_ea11b/2
  State_Px_1_SG_D_2_b2a07/1 -> Product_f0ef2/2
  Divide_4bdb1/1 -> Add_facde/2
  Constant_f0_dc763/1 -> Product_d0fc6/2
  Constant_-1_4eb38/1 -> Product_f0ef2/1
  Product_d0fc6/1 -> Add_d6f14/1
  Product_f0ef2/1 -> Divide_615c2/1
  Constant_T_w_8d456/1 -> Divide_615c2/2
  Divide_56502/1 -> Add_facde/1
  Add_d6f14/1 -> Divide_e6edd/1
  Product_5e1a3/1 -> Add_41ee7/2
  Constant_T_w_13561/1 -> Divide_e6edd/2
  Divide_615c2/1 -> Add_dc3fb/1
  State_Px_1_SG_D_2_ff7e4/1 -> Add_41ee7/1
  Divide_e6edd/1 -> Add_dc3fb/2
  Constant_-1_2becf/1 -> Product_28c6e/1
  Constant_T_2_9993e/1 -> Product_5e1a3/1
  Add_dc3fb/1 -> Product_5e1a3/2
  Product_ea11b/1 -> Divide_10a1c/1
  Constant_T_1_072f9/1 -> Divide_10a1c/2
  Add_41ee7/1 -> Divide_8e81c/1
  Constant_T_1_69240/1 -> Divide_8e81c/2
  Divide_10a1c/1 -> Add_faa06/1
  Divide_8e81c/1 -> Add_faa06/2
  Constant_T_4_abecd/1 -> Product_a6171/1
  Add_faa06/1 -> Product_a6171/2
  State_Px_3_SG_D_2_7c23f/1 -> Product_28c6e/2
  State_Px_2_SG_D_2_f11c4/1 -> Add_1629a/1
  Product_a6171/1 -> Add_1629a/2
  Product_28c6e/1 -> Divide_56502/1
  Constant_T_3_09de0/1 -> Divide_56502/2
  Constant_T_3_ac430/1 -> Divide_4bdb1/2
  Add_facde/1 -> Blockout_d_Px_3_SG_D_2_76e34/1

== system case9/Apparatus/SG_D_2/d_R_f_SG_D_2_block ==
  note: d_R_f_SG_D_2 in case9
      | $-\frac{R_{f,\mathrm{SG},D,2}-\frac{E_{\mathrm{fd},\mathrm{SG},D,2}\,K_{F}}{T_{F}}}{T_{F}}$
      | Automatically generated on 2025-10-31 19:35:03 .
  State_E_fd_SG_D_2_7e6fb : Inport
  State_R_f_SG_D_2_d286d : Inport  Port=2
  Constant_K_F_2c86a : Constant  Value=K_F
  Constant_T_F_234f8 : Constant  Value=T_F
  Constant_T_F_d5455 : Constant  Value=T_F
  Divide_68adb : Product  Inputs=*/
  Divide_cd4a0 : Product  Inputs=*/
  Product_14403 : Product
  Subtract_274f1 : Sum  Inputs=+-
  Blockout_d_R_f_SG_D_2_35db8 : Outport
  wires:
  Constant_T_F_d5455/1 -> Divide_cd4a0/2
  State_E_fd_SG_D_2_7e6fb/1 -> Product_14403/1
  Constant_K_F_2c86a/1 -> Product_14403/2
  State_R_f_SG_D_2_d286d/1 -> Subtract_274f1/2
  Product_14403/1 -> Divide_cd4a0/1
  Divide_cd4a0/1 -> Subtract_274f1/1
  Constant_T_F_234f8/1 -> Divide_68adb/2
  Subtract_274f1/1 -> Divide_68adb/1
  Divide_68adb/1 -> Blockout_d_R_f_SG_D_2_35db8/1

== system case9/Apparatus/SG_D_2/d_T_m_SG_D_2_block ==
  note: d_T_m_SG_D_2 in case9
      | $-\frac{T_{m,\mathrm{SG},D,2}-T_{0}+\frac{\mathrm{SpeedPara}\,\left(w_{\mathrm{SG},D,2}-w_{\mathrm{ref}}\right)}{2\,f_{0}\,\pi }}{T_{\mathrm{speed}}}$
      | Automatically generated on 2025-10-31 19:35:01 .
  State_w_SG_D_2_d76e3 : Inport
  State_T_m_SG_D_2_317ca : Inport  Port=2
  Add_0a679 : Sum
  Add_4c69b : Sum
  Constant_-1_9bcac : Constant  Value=-1
  Constant_2.0_85b40 : Constant  Value=2.0
  Constant_SpeedPara_27090 : Constant  Value=SpeedPara
  Constant_T_0_6d63b : Constant  Value=T_0
  Constant_T_speed_c998e : Constant  Value=T_speed
  Constant_f0_e24d7 : Constant  Value=f0
  Constant_pi_8b960 : Constant  Value=pi
  Constant_w_ref_6e01e : Constant  Value=w_ref
  Divide_6f321 : Product  Inputs=*/
  Divide_8242e : Product  Inputs=*/
  Product_77a54 : Product
  Product_97ea8 : Product
  Product_b397a : Product
  Product_e3b99 : Product
  Subtract_59fb3 : Sum  Inputs=+-
  Blockout_d_T_m_SG_D_2_6324f : Outport
  wires:
  Constant_pi_8b960/1 -> Product_b397a/2
  Constant_-1_9bcac/1 -> Product_97ea8/1
  Constant_w_ref_6e01e/1 -> Add_0a679/2
  State_w_SG_D_2_d76e3/1 -> Product_97ea8/2
  Product_97ea8/1 -> Add_0a679/1
  Add_4c69b/1 -> Subtract_59fb3/1
  Add_0a679/1 -> Product_77a54/2
  Constant_2.0_85b40/1 -> Product_b397a/1
  Constant_SpeedPara_27090/1 -> Product_77a54/1
  Product_b397a/1 -> Product_e3b99/1
  Constant_f0_e24d7/1 -> Product_e3b99/2
  Product_77a54/1 -> Divide_8242e/1
  Product_e3b99/1 -> Divide_8242e/2
  Divide_8242e/1 -> Add_4c69b/1
  Constant_T_0_6d63b/1 -> Add_4c69b/2
  State_T_m_SG_D_2_317ca/1 -> Subtract_59fb3/2
  Subtract_59fb3/1 -> Divide_6f321/1
  Constant_T_speed_c998e/1 -> Divide_6f321/2
  Divide_6f321/1 -> Blockout_d_T_m_SG_D_2_6324f/1

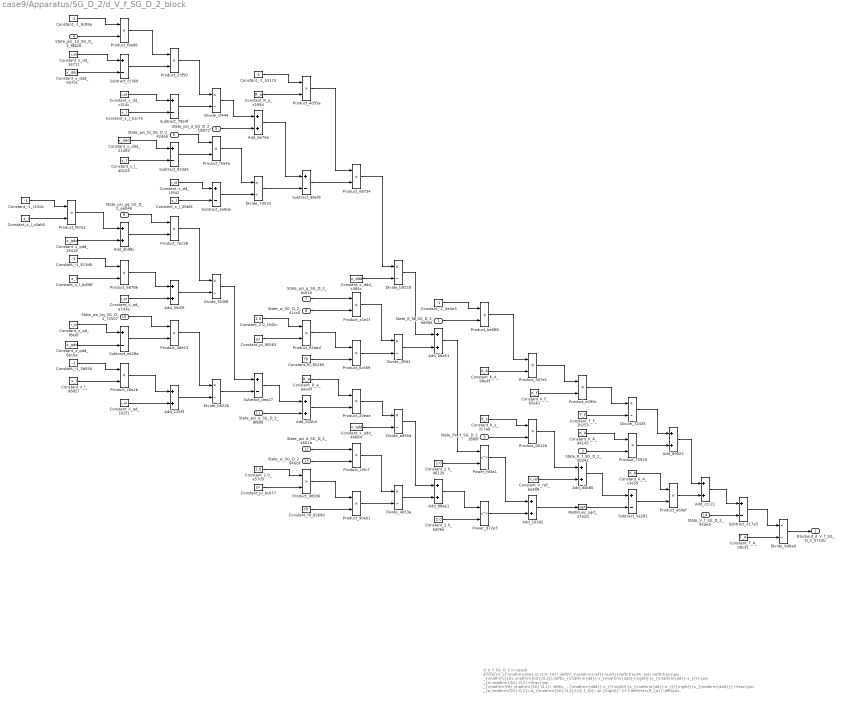
== system case9/Apparatus/SG_D_2/d_V_f_SG_D_2_block ==
  note: d_V_f_SG_D_2 in case9
      | $-\frac{V_{f,\mathrm{SG},D,2}-K_{A}\,\left(V_{\mathrm{ref}}-\sqrt{{\left(\frac{R_{a}\,\left(\frac{\psi _{\mathrm{1d},\mathrm{SG},D,2}\,\left(x_{\mathrm{dd}}-x_{\mathrm{ddd}}\right)}{x_{\mathrm{dd}}-x_{l}}-\psi _{d,\mathrm{SG},D,2}+\frac{\psi _{\mathrm{fd},\mathrm{SG},D,2}\,\left(x_{\mathrm{ddd}}-x_{l}\right)}{x_{\mathrm{dd}}-x_{l}}\right)}{x_{\mathrm{ddd}}}+\frac{\psi _{q,\mathrm{SG},D,2}\,w_{\mathrm{SG},D,2}}{2\,f_{0}\,\pi }\right)}^2+{\left(\frac{R_{a}\,\left(\psi _{q,\mathrm{SG},D,2}+\frac{\psi _{\mathrm{gq},\mathrm{SG},D,2}\,\left(x_{l}-x_{\mathrm{qdd}}\right)}{x_{l}-x_{\mathrm{qd}}}+\frac{\psi _{\mathrm{kq},\mathrm{SG},D,2}\,\left(x_{\mathrm{qd}}-x_{\mathrm{qdd}}\right)}{x_{l}-x_{\mathrm{qd}}}\right)}{x_{\mathrm{qdd}}}+\frac{\psi _{d,\mathrm{SG},D,2}\,w_{\mathrm{SG},D,2}}{2\,f_{0}\,\pi }\right)}^2}+K_{s}\,\mathrm{Px}_{3,\mathrm{SG},D,2}\right)-K_{A}\,R_{f,\mathrm{SG},D,2}+\frac{E_{\mathrm{fd},\mathrm{SG},D,2}\,K_{A}\,K_{F}}{T_{F}}}{T_{A}}$
      | Automatically generated on 2025-10-31 19:35:03 .
  State_E_fd_SG_D_2_9e906 : Inport
  State_R_f_SG_D_2_0b242 : Inport  Port=2
  State_Px_3_SG_D_2_18b0f : Inport  Port=3
  State_psi_1d_SG_D_2_f8826 : Inport  Port=4
  State_psi_d_SG_D_2_b0072 : Inport  Port=5
  State_psi_fd_SG_D_2_42d6b : Inport  Port=6
  State_psi_q_SG_D_2_6c610 : Inport  Port=7
  State_w_SG_D_2_41cc0 : Inport  Port=8
  State_psi_gq_SG_D_2_ee046 : Inport  Port=9
  State_psi_kq_SG_D_2_72507 : Inport  Port=10
  State_psi_q_SG_D_2_9f809 : Inport  Port=11
  State_psi_d_SG_D_2_4601a : Inport  Port=12
  State_w_SG_D_2_846cd : Inport  Port=13
  State_V_f_SG_D_2_42ae3 : Inport  Port=14
  Add_05d3f : Sum
  Add_126f3 : Sum
  Add_163d2 : Sum
  Add_625b4 : Sum
  Add_6a76e : Sum
  Add_88ae1 : Sum
  Add_89922 : Sum
  Add_bbe51 : Sum
  Add_ccc21 : Sum
  Add_d4b80 : Sum
  Add_db98c : Sum
  Constant_-1_0e4a3 : Constant  Value=-1
  Constant_-1_3b056 : Constant  Value=-1
  Constant_-1_913d6 : Constant  Value=-1
  Constant_-1_9c89a : Constant  Value=-1
  Constant_-1_b3115 : Constant  Value=-1
  Constant_-1_c15cb : Constant  Value=-1
  Constant_2.0_1fd2c : Constant  Value=2.0
  Constant_2.0_a57d3 : Constant  Value=2.0
  Constant_2.0_bd06e : Constant  Value=2.0
  Constant_2.0_d6120 : Constant  Value=2.0
  Constant_K_A_98e4f : Constant  Value=K_A
  Constant_K_A_c3e59 : Constant  Value=K_A
  Constant_K_A_d4142 : Constant  Value=K_A
  Constant_K_F_65eb1 : Constant  Value=K_F
  Constant_K_s_2c7ae : Constant  Value=K_s
  Constant_R_a_aaed3 : Constant  Value=R_a
  Constant_R_a_c595d : Constant  Value=R_a
  Constant_T_A_09c31 : Constant  Value=T_A
  Constant_T_F_1b253 : Constant  Value=T_F
  Constant_V_ref_be408 : Constant  Value=V_ref
  Constant_f0_8269d : Constant  Value=f0
  Constant_f0_85265 : Constant  Value=f0
  Constant_pi_90563 : Constant  Value=pi
  Constant_pi_bcb77 : Constant  Value=pi
  Constant_x_dd_16711 : Constant  Value=x_dd
  Constant_x_dd_1f942 : Constant  Value=x_dd
  Constant_x_dd_c314c : Constant  Value=x_dd
  Constant_x_ddd_0a7ce : Constant  Value=x_ddd
  Constant_x_ddd_21459 : Constant  Value=x_ddd
  Constant_x_ddd_c384c : Constant  Value=x_ddd
  Constant_x_l_00af4 : Constant  Value=x_l
  Constant_x_l_40103 : Constant  Value=x_l
  Constant_x_l_b1c7e : Constant  Value=x_l
  Constant_x_l_bd36f : Constant  Value=x_l
  Constant_x_l_c0ab5 : Constant  Value=x_l
  Constant_x_l_d8d27 : Constant  Value=x_l
  Constant_x_qd_102f1 : Constant  Value=x_qd
  Constant_x_qd_a7d3e : Constant  Value=x_qd
  Constant_x_qd_f8e0f : Constant  Value=x_qd
  Constant_x_qdd_19418 : Constant  Value=x_qdd
  Constant_x_qdd_46664 : Constant  Value=x_qdd
  Constant_x_qdd_6ec6a : Constant  Value=x_qdd
  Divide_2ffd1 : Product  Inputs=*/
  Divide_4653a : Product  Inputs=*/
  Divide_6d0a0 : Product  Inputs=*/
  Divide_72435 : Product  Inputs=*/
  Divide_7d533 : Product  Inputs=*/
  Divide_ad95d : Product  Inputs=*/
  Divide_b622b : Product  Inputs=*/
  Divide_b9228 : Product  Inputs=*/
  Divide_cf444 : Product  Inputs=*/
  Divide_f2008 : Product  Inputs=*/
  MathFunc_sqrt_27e2d : Sqrt
  Power_972e3 : Math  Operator=pow
  Power_fd4a1 : Math  Operator=pow
  Product_20eaa : Product
  Product_23f50 : Product
  Product_307e1 : Product
  Product_48e13 : Product
  Product_4d35a : Product
  Product_68786 : Product
  Product_6c469 : Product
  Product_75929 : Product
  Product_7ec58 : Product
  Product_90eb1 : Product
  Product_92abd : Product
  Product_be088 : Product
  Product_c1e1f : Product
  Product_c5fc7 : Product
  Product_c8a2b : Product
  Product_d012b : Product
  Product_d8936 : Product
  Product_e290c : Product
  Product_e69ef : Product
  Product_e8734 : Product
  Product_f5a4a : Product
  Product_f67a1 : Product
  Product_f9a86 : Product
  Subtract_0a281 : Sum  Inputs=+-
  Subtract_2e8de : Sum  Inputs=+-
  Subtract_68ef8 : Sum  Inputs=+-
  Subtract_7954f : Sum  Inputs=+-
  Subtract_923d5 : Sum  Inputs=+-
  Subtract_cc369 : Sum  Inputs=+-
  Subtract_dea27 : Sum  Inputs=+-
  Subtract_e17a5 : Sum  Inputs=+-
  Subtract_e628a : Sum  Inputs=+-
  Blockout_d_V_f_SG_D_2_0715b : Outport
  wires:
  Constant_-1_9c89a/1 -> Product_f9a86/1
  Constant_2.0_1fd2c/1 -> Product_92abd/1
  Constant_-1_c15cb/1 -> Product_f67a1/1
  Product_92abd/1 -> Product_6c469/1
  Product_f67a1/1 -> Add_db98c/1
  Constant_x_l_d8d27/1 -> Product_c8a2b/2
  Constant_x_l_c0ab5/1 -> Product_f67a1/2
  State_psi_1d_SG_D_2_f8826/1 -> Product_f9a86/2
  Constant_x_l_00af4/1 -> Subtract_2e8de/2
  Constant_x_dd_16711/1 -> Subtract_cc369/1
  Product_20eaa/1 -> Divide_ad95d/1
  Constant_x_ddd_0a7ce/1 -> Subtract_cc369/2
  Constant_x_qd_102f1/1 -> Add_126f3/2
  Add_db98c/1 -> Product_7ec58/2
  Constant_x_qdd_19418/1 -> Add_db98c/2
  Constant_-1_913d6/1 -> Product_68786/1
  Constant_x_dd_1f942/1 -> Subtract_2e8de/1
  Subtract_dea27/1 -> Add_625b4/1
  Power_fd4a1/1 -> Add_163d2/1
  Constant_x_l_bd36f/1 -> Product_68786/2
  Constant_2.0_a57d3/1 -> Product_d8936/1
  Constant_x_qd_f8e0f/1 -> Subtract_e628a/1
  Constant_pi_bcb77/1 -> Product_d8936/2
  Subtract_68ef8/1 -> Product_e8734/2
  Constant_x_qdd_6ec6a/1 -> Subtract_e628a/2
  State_psi_fd_SG_D_2_42d6b/1 -> Product_f5a4a/1
  Constant_-1_3b056/1 -> Product_c8a2b/1
  Product_f9a86/1 -> Product_23f50/1
  State_w_SG_D_2_846cd/1 -> Product_c5fc7/2
  Subtract_cc369/1 -> Product_23f50/2
  Constant_x_dd_c314c/1 -> Subtract_7954f/1
  State_psi_q_SG_D_2_9f809/1 -> Add_625b4/2
  State_w_SG_D_2_41cc0/1 -> Product_c1e1f/2
  Subtract_923d5/1 -> Product_f5a4a/2
  Constant_x_l_b1c7e/1 -> Subtract_7954f/2
  Add_89922/1 -> Add_ccc21/1
  Constant_x_ddd_21459/1 -> Subtract_923d5/1
  Constant_x_l_40103/1 -> Subtract_923d5/2
  State_psi_gq_SG_D_2_ee046/1 -> Product_7ec58/1
  Product_68786/1 -> Add_05d3f/1
  Subtract_2e8de/1 -> Divide_7d533/2
  Constant_x_qd_a7d3e/1 -> Add_05d3f/2
  Product_c1e1f/1 -> Divide_2ffd1/1
  State_psi_kq_SG_D_2_72507/1 -> Product_48e13/1
  Subtract_e628a/1 -> Product_48e13/2
  Product_f5a4a/1 -> Divide_7d533/1
  State_V_f_SG_D_2_42ae3/1 -> Subtract_e17a5/2
  Product_c8a2b/1 -> Add_126f3/1
  Product_23f50/1 -> Divide_cf444/1
  Divide_f2008/1 -> Subtract_dea27/1
  Subtract_7954f/1 -> Divide_cf444/2
  Product_7ec58/1 -> Divide_f2008/1
  Add_05d3f/1 -> Divide_f2008/2
  Product_48e13/1 -> Divide_b622b/1
  Divide_7d533/1 -> Subtract_68ef8/2
  Constant_f0_85265/1 -> Product_6c469/2
  Add_126f3/1 -> Divide_b622b/2
  Divide_cf444/1 -> Add_6a76e/1
  State_psi_d_SG_D_2_b0072/1 -> Add_6a76e/2
  Divide_b622b/1 -> Subtract_dea27/2
  Constant_-1_b3115/1 -> Product_4d35a/1
  Constant_R_a_c595d/1 -> Product_4d35a/2
  Constant_f0_8269d/1 -> Product_90eb1/2
  Add_6a76e/1 -> Subtract_68ef8/1
  Product_4d35a/1 -> Product_e8734/1
  Constant_pi_90563/1 -> Product_92abd/2
  State_psi_q_SG_D_2_6c610/1 -> Product_c1e1f/1
  Constant_R_a_aaed3/1 -> Product_20eaa/1
  State_E_fd_SG_D_2_9e906/1 -> Product_be088/2
  Add_625b4/1 -> Product_20eaa/2
  State_psi_d_SG_D_2_4601a/1 -> Product_c5fc7/1
  Product_d8936/1 -> Product_90eb1/1
  Product_e8734/1 -> Divide_b9228/1
  Constant_x_ddd_c384c/1 -> Divide_b9228/2
  Product_6c469/1 -> Divide_2ffd1/2
  Constant_x_qdd_46664/1 -> Divide_ad95d/2
  Product_c5fc7/1 -> Divide_4653a/1
  Product_90eb1/1 -> Divide_4653a/2
  Divide_b9228/1 -> Add_bbe51/1
  Divide_2ffd1/1 -> Add_bbe51/2
  Divide_ad95d/1 -> Add_88ae1/1
  Divide_4653a/1 -> Add_88ae1/2
  Constant_-1_0e4a3/1 -> Product_be088/1
  Add_bbe51/1 -> Power_fd4a1/1
  Constant_2.0_d6120/1 -> Power_fd4a1/2
  Add_88ae1/1 -> Power_972e3/1
  Constant_2.0_bd06e/1 -> Power_972e3/2
  Product_be088/1 -> Product_307e1/1
  Constant_K_A_98e4f/1 -> Product_307e1/2
  Constant_K_s_2c7ae/1 -> Product_d012b/1
  State_Px_3_SG_D_2_18b0f/1 -> Product_d012b/2
  Power_972e3/1 -> Add_163d2/2
  Product_307e1/1 -> Product_e290c/1
  Constant_K_F_65eb1/1 -> Product_e290c/2
  Product_d012b/1 -> Add_d4b80/1
  Constant_V_ref_be408/1 -> Add_d4b80/2
  Add_163d2/1 -> MathFunc_sqrt_27e2d/1
  Product_e290c/1 -> Divide_72435/1
  Constant_T_F_1b253/1 -> Divide_72435/2
  Constant_K_A_d4142/1 -> Product_75929/1
  State_R_f_SG_D_2_0b242/1 -> Product_75929/2
  Add_d4b80/1 -> Subtract_0a281/1
  MathFunc_sqrt_27e2d/1 -> Subtract_0a281/2
  Divide_72435/1 -> Add_89922/1
  Product_75929/1 -> Add_89922/2
  Constant_K_A_c3e59/1 -> Product_e69ef/1
  Subtract_0a281/1 -> Product_e69ef/2
  Product_e69ef/1 -> Add_ccc21/2
  Add_ccc21/1 -> Subtract_e17a5/1
  Subtract_e17a5/1 -> Divide_6d0a0/1
  Constant_T_A_09c31/1 -> Divide_6d0a0/2
  Divide_6d0a0/1 -> Blockout_d_V_f_SG_D_2_0715b/1
